simulink model "modelMCC"  (R2018a)
settings: Solver=VariableStepAuto  StartTime=0.0  StopTime=10.0  RelTol=1e-3
settings Model: Creator=ilier  LastModifiedBy=ilier

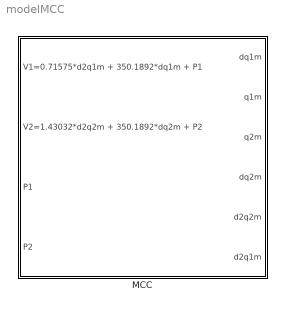
== system modelMCC ==
  MCC : Subsystem

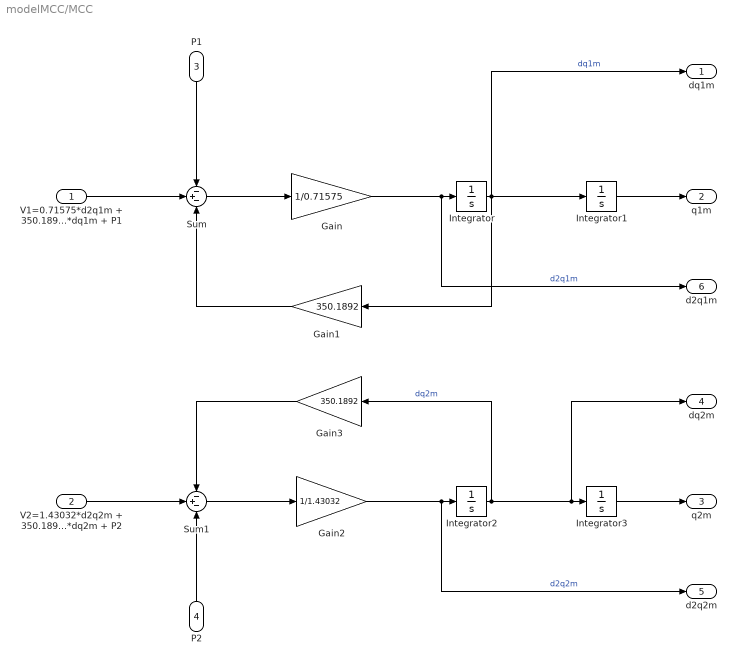
== system modelMCC/MCC ==
  V1=0.71575*d2q1m + 350.1892*dq1m + P1 : Inport
  V2=1.43032*d2q2m + 350.1892*dq2m + P2 : Inport  Port=2
  P1 : Inport  Port=3
  P2 : Inport  Port=4
  Gain : Gain  Gain=1/0.71575
  Gain1 : Gain  Gain=350.1892
  Gain2 : Gain  Gain=1/1.43032
  Gain3 : Gain  Gain=350.1892
  Integrator{,1..3} (4 alike) : Integrator
  Sum : Sum  Inputs=-+-
  Sum1 : Sum  Inputs=-+-
  dq1m : Outport
  q1m : Outport  Port=2
  q2m : Outport  Port=3
  dq2m : Outport  Port=4
  d2q2m : Outport  Port=5
  d2q1m : Outport  Port=6
  wires:
  Integrator3/1 -> q2m/1
  Integrator/1 -> dq1m/1, Integrator1/1, Gain1/1  "dq1m"
  P1/1 -> Sum/1
  V2=1.43032*d2q2m + 350.1892*dq2m + P2/1 -> Sum1/2
  Integrator2/1 -> Gain3/1, dq2m/1, Integrator3/1  "dq2m"
  Gain1/1 -> Sum/3
  V1=0.71575*d2q1m + 350.1892*dq1m + P1/1 -> Sum/2
  Gain/1 -> d2q1m/1, Integrator/1  "d2q1m"
  Integrator1/1 -> q1m/1
  Sum/1 -> Gain/1
  Gain2/1 -> d2q2m/1, Integrator2/1  "d2q2m"
  Gain3/1 -> Sum1/1
  Sum1/1 -> Gain2/1
  P2/1 -> Sum1/3
